simulink model "flyback"  (R2021a)
settings: Solver=FixedStepDiscrete  StartTime=0.0  StopTime=0.020  FixedStep=Ts/1000  RelTol=1e-3
values from neighbouring files (symbols this model uses):
  C = 100e-6    (= 0.0001)    [flyback_params.m]
  D = V/(V + N*Vg)    (= 0.333333333333)    [flyback_params.m]
  Lm = 250e-6    (= 0.00025)    [flyback_params.m]
  N = 1/2    (= 0.5)    [flyback_params.m]
  R = V/ Iout    (= 28.125)    [flyback_params.m]
  Ts = 1/fsw    (= 1e-05)    [flyback_params.m]
  Vg = 48    [flyback_params.m]
libraries: spsGroundLib x2, spsSeriesRLCBranchLib x2, spsCurrentMeasurementLib x1, spsDCVoltageSourceLib x1, spsDiodeLib x1, spsIdealSwitchLib x1, spsLinearTransformerLib x1, spsMultimeterLib x1, spsPWMGeneratorDCDCLib x1, spsVoltageMeasurementLib x1, spspowerguiLib x1
settings Model: Creator=yoshi  LastModifiedBy=yoshi

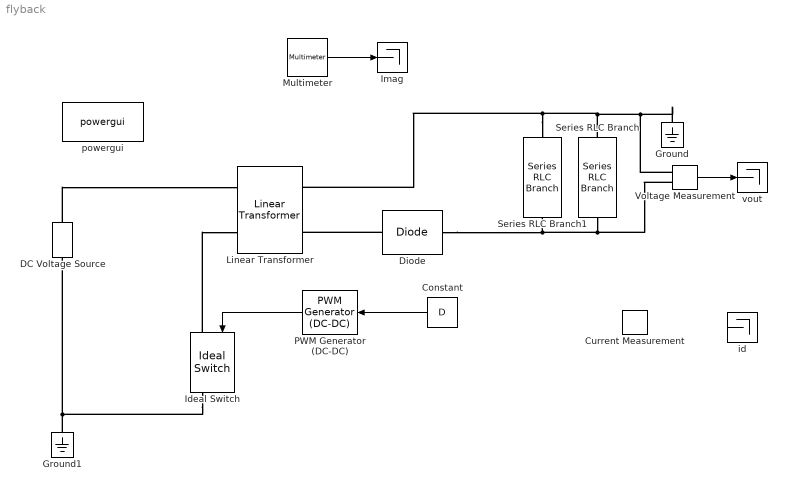
== system flyback ==
  Constant : Constant  Value=D
  Current Measurement : spsCurrentMeasurementLib/Current Measurement  PhasorSimulation=off  OutputType=Complex  PSBequivalent=0
  DC Voltage Source : spsDCVoltageSourceLib/DC Voltage Source  Amplitude=Vg  Measurements=None
  Diode : spsDiodeLib/Diode  Ron=1e-6  Lon=0  Vf=0  IC=0  UseSnubber=0  Rs=500  Cs=0  Measurements=off
  Ground : spsGroundLib/Ground  LConnTagsString=a
  Ground1 : spsGroundLib/Ground  LConnTagsString=a
  Ideal Switch : spsIdealSwitchLib/Ideal Switch  Ron=0.001  Lon=0  IC=0  Rs=1e5  Cs=inf  Measurements=on
  Imag : Terminator
  Linear Transformer : spsLinearTransformerLib/Linear Transformer  UNITS=SI  NominalPower=[ 250e6 60 ]  winding1=[7.35e5 0 0]  winding2=[N*7.35e5 0 0]  ThreeWindings=off  winding3=[3.15e+05 0.7938 0.084225]  RmLm=[1e6 Lm]  Measurements=Magnetization current  DataType=on
  Multimeter : spsMultimeterLib/Multimeter  PhasorSimulation=off  OutputType=Complex  sel=2  L=3  Gain=1  yselected={'Imag: Linear Transformer'};  PSBOutputType=1  PSBequivalent=0  AxesSetting=[0,0.1,-100,100]  Display=0  SavedBlockNames=-11
  PWM Generator (DC-DC) : spsPWMGeneratorDCDCLib/PWM Generator (DC-DC)  Fsw=fsw  Ts=0
  Series RLC Branch : spsSeriesRLCBranchLib/Series RLC Branch  LConnTagsString=__new0  RConnTagsString=__new0  BranchType=R  Resistance=R  Inductance=1e-3  SetiL0=off  InitialCurrent=0  Capacitance=1e-6  Setx0=off  InitialVoltage=0  Measurements=None
  Series RLC Branch1 : spsSeriesRLCBranchLib/Series RLC Branch  LConnTagsString=__new0  RConnTagsString=__new0  BranchType=C  Resistance=1  Inductance=1e-3  SetiL0=off  InitialCurrent=0  Capacitance=C  Setx0=off  InitialVoltage=0  Measurements=None
  Voltage Measurement : spsVoltageMeasurementLib/Voltage Measurement  PhasorSimulation=off  OutputType=Complex  PSBequivalent=0
  id : Terminator
  powergui : spspowerguiLib/powergui  Priority=1  SimulationMode=Discrete  SampleTime=Ts/1000  frequency=60  Iterations=50  frequencyindice=0  Pbase=100e6  ErrMax=1e-4  UnitsV=kV  UnitsW=MW  buscounter=0  FunctionMessages=off  echomessages=off  EnableUseOfTLC=off  CurrentSourceSwitches=off  DisableSnubberDevices=off  DisableRonSwitches=off  DisableVfSwitches=off  DisplayEquations=off  AutomaticDiscreteSolvers=off  SolverType=Tustin/Backward Euler (TBE)  Interpol=off  ExternalGateDelay=off  methode=off  Ts=100  x0status=blocks  SPID=on  SwTol=0  HookPort=off  NonlinearTolerance=1e-4  nMaxIteration=100  ContinueOnMaxIteration=off  RestoreLinks=warning  ResistiveCurrentMeasurement=off  Frange=[0:2:500]  Ylog=off  Xlog=on  ShowGrid=off  save=off  variable=ZData  structure=0  ZoomFFT=off  StartTime=0.0  cycles=1  DisplayStyle=1  fundamental=60  FreqAxis=off  MaxFrequency=1000  frequencyindicesteady=1  RmsSteady=1  display=off
  vout : Terminator
  wires:
  Voltage Measurement/1 -> vout/1
  PWM Generator (DC-DC)/1 -> Ideal Switch/1
  Constant/1 -> PWM Generator (DC-DC)/1
  Multimeter/1 -> Imag/1
  connections:
  Ideal Switch/LConn1 -- Linear Transformer/LConn2
  Ideal Switch/RConn1 -- Ground1/LConn1 -- DC Voltage Source/LConn1
  DC Voltage Source/RConn1 -- Linear Transformer/LConn1
  Diode/RConn1 -- Voltage Measurement/LConn1 -- Series RLC Branch/RConn1 -- Series RLC Branch1/LConn1
  Series RLC Branch1/RConn1 -- Ground/LConn1 -- Voltage Measurement/LConn2 -- Series RLC Branch/LConn1 -- Linear Transformer/RConn1
  Diode/LConn1 -- Linear Transformer/RConn2
